simulink model "pgct_stact"  (R2019a)
settings: Solver=VariableStepAuto  StartTime=0.0  StopTime=10.0  RelTol=1e-3
libraries: simulink x1
settings Model: Creator=rosha  LastModifiedBy=rosha

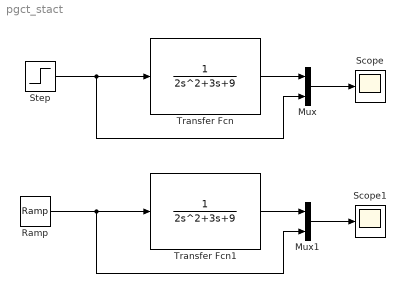
== system pgct_stact ==
  Mux : Mux  Inputs=2
  Mux1 : Mux  Inputs=2
  Ramp : simulink/Sources/Ramp  slope=1  start=0  InitialOutput=0
  Scope : Scope
  Scope1 : Scope
  Step : Step  SampleTime=0
  Transfer Fcn : TransferFcn  Denominator=[2 3 9]
  Transfer Fcn1 : TransferFcn  Denominator=[2 3 9]
  wires:
  Step/1 -> Mux/2, Transfer Fcn/1
  Transfer Fcn/1 -> Mux/1
  Mux/1 -> Scope/1
  Ramp/1 -> Mux1/2, Transfer Fcn1/1
  Transfer Fcn1/1 -> Mux1/1
  Mux1/1 -> Scope1/1
